simulink model "Motorcontrol"  (R2025b)
settings: Solver=VariableStepAuto  StartTime=0.0  StopTime=800  RelTol=1e-3
values from neighbouring files (symbols this model uses):
  A_hotend = lambda_dom    [fred_lqr_hotend_FIX.m]
  B_hotend = 1 - lambda_dom    [fred_lqr_hotend_FIX.m]
  C_hotend = DC_gain    [fred_lqr_hotend_FIX.m]
  Nbar_hotend = rscale_discrete(A_hotend, B_hotend, C_hotend, D_hotend, K_hotend)    [fred_lqr_hotend_FIX.m]
undefined symbols (not defined in the file or in its folder): K_hotend
settings Model: Creator=kenom  LastModifiedBy=MATEO

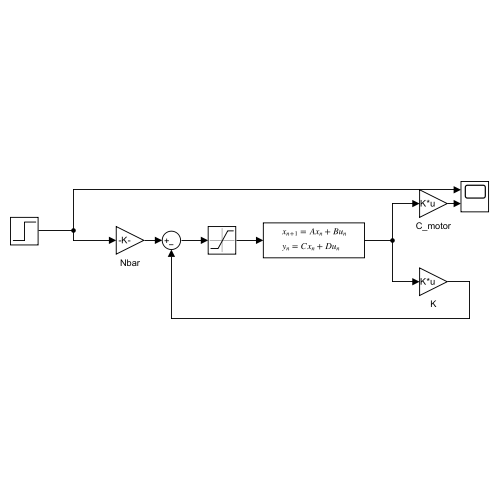
[thumbnail: Simulink's stored preview of the top-level diagram]
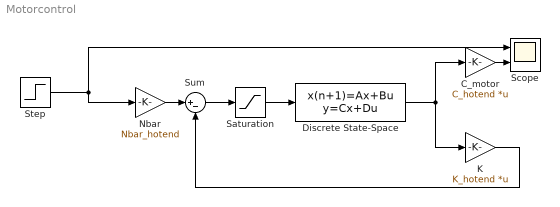
== system Motorcontrol ==
  C_motor : Gain  Gain=C_hotend  Multiplication=Matrix(K*u)
  Discrete State-Space : DiscreteStateSpace  A=A_hotend  B=B_hotend  C=eye(size(A_hotend))  D=zeros(size(A_hotend,1),1)  SampleTime=0.1
  K : Gain  Gain=K_hotend  Multiplication=Matrix(K*u)
  Nbar : Gain  Gain=Nbar_hotend
  Saturation : Saturate  UpperLimit=255  LowerLimit=-255
  Scope : Scope  NumInputPorts=2
      settings: ActiveDisplayYMinimum=-4.3945210994805537  ActiveDisplayYMaximum=39.550689895324993
  Step : Step  Time=0  After=200  SampleTime=0.1
  Sum : Sum  Inputs=|+-
  wires:
  Nbar/1 -> Sum/1
  Sum/1 -> Saturation/1
  Saturation/1 -> Discrete State-Space/1
  K/1 -> Sum/2
  Step/1 -> Nbar/1, Scope/1
  Discrete State-Space/1 -> C_motor/1, K/1
  C_motor/1 -> Scope/2
